simulink model "Quadroto_Outer_Loop"  (Simulink 7.6)
settings: Solver=FixedStepDiscrete  StartTime=0.0  StopTime=10.0  FixedStep=0.01  RelTol=1e-3
libraries: passive_control x1
settings Model: Creator=jporter  LastModifiedBy=Administrator
settings DataIOCC: LimitDataPoints=off  SaveOutput=off  SignalLogging=off  DSMLogging=off  SaveTime=off
settings OptimizationCC: InlineParams=on  EnhancedBackFolding=on  PassReuseOutputArgsAs=Individual arguments  OptimizeModelRefInitCode=on
settings HardwareCC: ProdLargestAtomicInteger=Long  ProdLargestAtomicFloat=Float  ProdIntDivRoundTo=Floor  ProdEndianess=LittleEndian  ProdHWDeviceType=ARM Compatible->ARM 7  TargetLargestAtomicInteger=Long  TargetLargestAtomicFloat=Float  TargetIntDivRoundTo=Floor  TargetEndianess=LittleEndian  TargetHWDeviceType=ARM Compatible->ARM 7
settings RTWCC: SystemTargetFile=ert.tlc  GenCodeOnly=on  TemplateMakefile=ert_default_tmf  Description=Real-Time Workshop Embedded Coder  GenerateReport=on  ProcessScript=ert_make_rtw_hook  IncludeHyperlinkInReport=on  LaunchReport=on  GenerateTraceReportSl=on  GenerateTraceReportEml=on  RTWCompilerOptimization=On  CheckMdlBeforeBuild=Warning
settings CodeAppCC: IgnoreCustomStorageClasses=off
settings ERTTargetCC: MultiwordLength=2048  GenerateSampleERTMain=on  CombineSignalStateStructs=on  MultiInstanceERTCode=on  SupportComplex=off  MultiInstanceErrorCode=Warning  ERTCustomFileTemplate=example_file_process.tlc

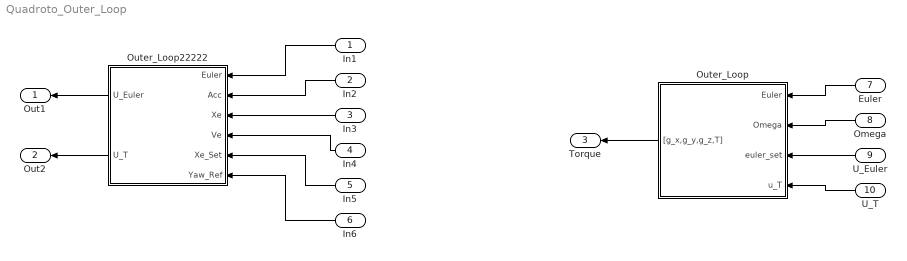
== system Quadroto_Outer_Loop ==
  In1 : Inport  OutDataTypeStr=single  PortDimensions=[3]
  In2 : Inport  Port=2  OutDataTypeStr=single  PortDimensions=[3]
  In3 : Inport  Port=3  OutDataTypeStr=single  PortDimensions=[3]
  In4 : Inport  Port=4  OutDataTypeStr=single  PortDimensions=[3]
  In5 : Inport  Port=5  OutDataTypeStr=single  PortDimensions=[3]
  In6 : Inport  Port=6  OutDataTypeStr=single  PortDimensions=[1]
  Euler : Inport  Port=7  OutDataTypeStr=single  PortDimensions=[3]
  Omega : Inport  Port=8  OutDataTypeStr=single  PortDimensions=[3]
  U_Euler : Inport  Port=9  OutDataTypeStr=single  PortDimensions=[3]
  U_T : Inport  Port=10  OutDataTypeStr=single  PortDimensions=[1]
  Outer_Loop : Subsystem
  Outer_Loop22222 : Subsystem
  Out1 : Outport
  Out2 : Outport  Port=2
  Torque : Outport  Port=3
  wires:
  In1/1 -> Outer_Loop22222/1(Euler)
  In2/1 -> Outer_Loop22222/2(Acc)
  In3/1 -> Outer_Loop22222/3(Xe)
  In4/1 -> Outer_Loop22222/4(Ve)
  In5/1 -> Outer_Loop22222/5(Xe_Set)
  In6/1 -> Outer_Loop22222/6(Yaw_Ref)
  Outer_Loop22222/1(U_Euler) -> Out1/1
  Outer_Loop22222/2(U_T) -> Out2/1
  Euler/1 -> Outer_Loop/1(Euler)
  Omega/1 -> Outer_Loop/2(Omega)
  U_Euler/1 -> Outer_Loop/3(euler_set)
  U_T/1 -> Outer_Loop/4(u_T)
  Outer_Loop/1("[g_x,g_y,g_z,T]") -> Torque/1

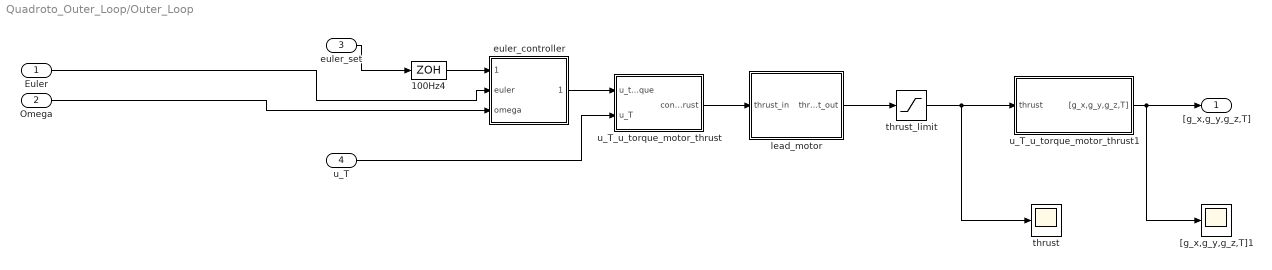
== system Quadroto_Outer_Loop/Outer_Loop ==
  Euler : Inport  OutDataTypeStr=single
  Omega : Inport  Port=2  OutDataTypeStr=single
  euler_set : Inport  Port=3  OutDataTypeStr=single
  u_T : Inport  Port=4  OutDataTypeStr=single
  100Hz4 : ZeroOrderHold  SampleTime=.01
  "[g_x,g_y,g_z,T]1" : Scope
      settings: TimeRange=100  YMin=3  YMax=10  SaveName=thrust_data10  MaxDataPoints=50000
  euler_controller : Subsystem  mask{K=1, K_e=2*7.5/.65, K_o=.5*.25, I=diag([2.32,2.32,4.41]*1e-3), T_max=3.7*1, delta=.343/2, K_t=1.5e-9/6.11e-8}
      mask prompts: K "Loop Gain [K]:"; K_e "Euler Gain [K_e]:"; K_o "Omega Gain [K_o]:"; I "Inertia Matrix [I]:"; T_max "Max Rotor Thrust [T_max] (N):"; delta "Distance from CG to rotor [delta] (m):"; K_t "z-torque gain [K_t]:"
      mask init:
      | I=[I(1,1),I(2,2),I(3,3)];
      | I_norm=I*(1/min(I))
  lead_motor : Subsystem  mask{tau_motor=1/20, Ts=1/100, m=.489}
      mask prompts: m "mass of quadrotor (kg) [m]"
      mask init:
      | Hs=tf([tau_motor, 1],[Ts/pi, 1]);
      | Hz=ipesh_transform(Hs,Ts)
      | Hz.num{1}
      | Hz.den{1}
      | %a=1/tau_motor;
      | %b=pi/t_s;
      | %T=t_s;
      | %num1=b*(1-exp(-b*T))+a*(b*T-1+exp(-b*T));
      | %num2=-b*(1-exp(-b*T))+a*(1-exp(-b*T)-b*T*exp(-b*T));
      | %den1=a*b;
      | %den2=-a*b*exp(-b*T);
      | %num=[num1 num2];
      | %den=[den1 den2];
      | %Hz=tf(num,den,T);
      | %[y,t]=step(Hz);
      | %k_ss=(1/y(length(y)));
      | %num=k_ss*num;
      | %lead_a_1=single(-den(2)/den(1))
      | %lead_b_1=single(num(2)/den(1))
      | %lead_b_2=single(num(1)/den(1))
      | %Hz=k_ss*Hz
      | %bode(Hz);
  thrust : Scope
      settings: TimeRange=100  YMin=3  YMax=10  SaveName=thrust_data  MaxDataPoints=50000
  thrust_limit : Saturate  UpperLimit=3.7*ones(4,1)  LowerLimit=0*ones(4,1)  OutDataTypeStr=single
  u_T_u_torque_motor_thrust : Subsystem  mask{dx=1*.343/2, K_torque=1.5e-9/6.11e-8}
      mask prompts: dx "X distance of motor from CG [dx](meters):"; K_torque "Ktorque [K_torque]:"
      mask init:
      | M=[0 -dx 0 dx;
      |    dx 0 -dx 0;
      |    -K_torque K_torque -K_torque K_torque;
      |    1 1 1 1];
      | Mi=single(inv(M))
  u_T_u_torque_motor_thrust1 : Subsystem  mask{delta=.343/2, K_t=1.5e-9/6.11e-8, T_max=3.7, Ts=.01}
      mask prompts: delta "X distance of motor from CG [delta](meters):"; K_t "Ktorque [K_torque]:"; T_max "Max Rotor Thrust [T_max]:"; Ts "Sample Time [Ts]:"
      mask init:
      | M=single([0 -delta 0 delta;
      |    delta 0 -delta 0;
      |    -K_t K_t -K_t K_t;
      |    1 1 1 1]);
  "[g_x,g_y,g_z,T]" : Outport
  wires:
  euler_set/1 -> 100Hz4/1
  u_T/1 -> u_T_u_torque_motor_thrust/2(u_T)
  euler_controller/1(u_torque) -> u_T_u_torque_motor_thrust/1(u_torque)
  thrust_limit/1 -> thrust/1, u_T_u_torque_motor_thrust1/1(thrust)
  u_T_u_torque_motor_thrust/1(cont_motor_thrust) -> lead_motor/1(thrust_in)
  lead_motor/1(thrust_out) -> thrust_limit/1
  u_T_u_torque_motor_thrust1/1("[g_x,g_y,g_z,T]") -> "[g_x,g_y,g_z,T]"/1, "[g_x,g_y,g_z,T]1"/1
  100Hz4/1 -> euler_controller/1(euler_set)
  Euler/1 -> euler_controller/2(euler)
  Omega/1 -> euler_controller/3(omega)

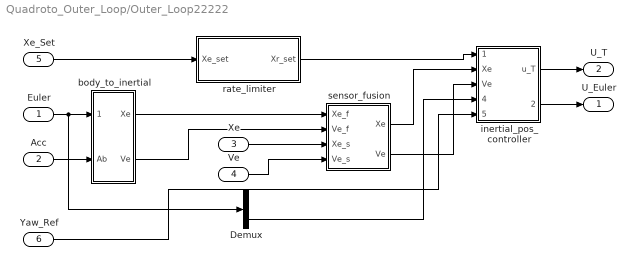
== system Quadroto_Outer_Loop/Outer_Loop22222 ==
  Euler : Inport  OutDataTypeStr=single  PortDimensions=[3]
  Acc : Inport  Port=2  OutDataTypeStr=single  PortDimensions=[3]
  Xe : Inport  Port=3  OutDataTypeStr=single  PortDimensions=[3]
  Ve : Inport  Port=4  OutDataTypeStr=single  PortDimensions=[3]
  Xe_Set : Inport  Port=5  OutDataTypeStr=single  PortDimensions=[3]
  Yaw_Ref : Inport  Port=6  OutDataTypeStr=single  PortDimensions=[1]
  Demux : Demux  Outputs=3
  body_to_inertial : Subsystem
  inertial_pos_controller : Subsystem
  rate_limiter : Subsystem  mask{wn=2*pi, zeta=0.9, Vmax=2, T=0.01}
      mask prompts: wn "omega_n"; Vmax "Max velocity"; T "Sample time"
      mask init:
      | Hs=tf([wn^2],[1,2*zeta*wn,wn^2]);
      | Hz=ipesh_transform(Hs,T);
  sensor_fusion : Subsystem  mask{tau=.1, Ts=.01, Ts_gps=.1}
      mask prompts: tau "low-pass time constant (sec) [tau]"; Ts "Sample time [Ts]"; Ts_gps "GPS Sample Time [Ts_gps]"
  U_Euler : Outport  OutDataTypeStr=single  PortDimensions=[3]
  U_T : Outport  Port=2  OutDataTypeStr=single  PortDimensions=[1]
  wires:
  Xe_Set/1 -> rate_limiter/1(Xe_set)
  inertial_pos_controller/1(u_T) -> U_T/1
  inertial_pos_controller/2(u_euler) -> U_Euler/1
  Euler/1 -> body_to_inertial/1(euler), Demux/1
  Acc/1 -> body_to_inertial/2(Ab)
  sensor_fusion/1(Xe) -> inertial_pos_controller/2(Xe)
  sensor_fusion/2(Ve) -> inertial_pos_controller/3(Ve)
  body_to_inertial/1(Xe) -> sensor_fusion/1(Xe_f)
  body_to_inertial/2(Ve) -> sensor_fusion/2(Ve_f)
  Xe/1 -> sensor_fusion/3(Xe_s)
  Ve/1 -> sensor_fusion/4(Ve_s)
  rate_limiter/1(Xr_set) -> inertial_pos_controller/1(Xe_set)
  Demux/3 -> inertial_pos_controller/4(Yaw_actual)
  Yaw_Ref/1 -> inertial_pos_controller/5(Yaw_set)

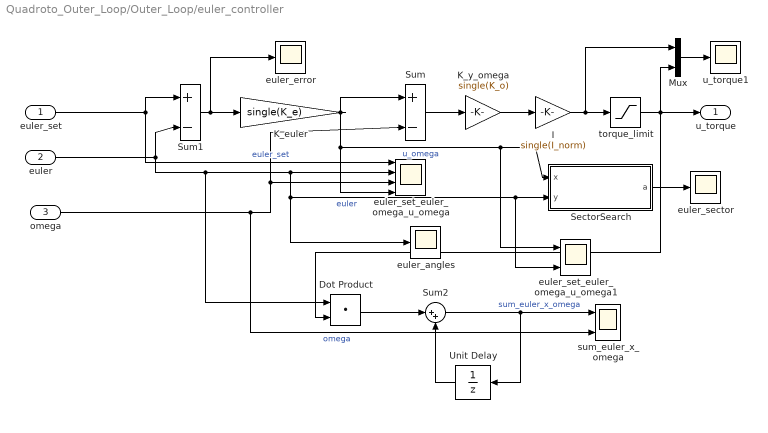
== system Quadroto_Outer_Loop/Outer_Loop/euler_controller ==
  euler_set : Inport
  euler : Inport  Port=2
  omega : Inport  Port=3
  Dot Product : DotProduct  InputSameDT=on  OutDataTypeStr=Inherit: Inherit via internal rule
  I : Gain  Gain=single(I_norm)  OutDataTypeStr=single
  K_euler : Gain  Gain=single(K_e)
  K_y_omega : Gain  Gain=single(K_o)  OutDataTypeStr=single
  Mux : Mux  Inputs=2
  SectorSearch : Subsystem  AncestorBlock=passive_control/SectorSearch
  Sum : Sum  Inputs=|+-  AccumDataTypeStr=single
  Sum1 : Sum  Inputs=|+-  AccumDataTypeStr=single
  Sum2 : Sum  Inputs=|++
  Unit Delay : UnitDelay  SampleTime=-1
  euler_angles : Scope
      settings: TimeRange=80  YMin=-1.1  YMax=1.1  SaveName=euler_data  MaxDataPoints=50000
  euler_error : Scope
      settings: TimeRange=80  YMin=-0.011  YMax=0.011  SaveName=euler_data1  MaxDataPoints=50000
  euler_sector : Scope
      settings: TimeRange=80  YMin=-1  YMax=1  SaveName=euler_sector_data  MaxDataPoints=50000
  euler_set_euler_omega_u_omega : Scope  NumInputPorts=4
      settings: YMin=-7~-7~-0.3~-0.3  YMax=1~1~0.3~0.3  SaveName=ScopeData8
  euler_set_euler_omega_u_omega1 : Scope  NumInputPorts=2
      settings: YMin=-7~-7  YMax=1~1  SaveName=ScopeData5  Decimation=10
  sum_euler_x_omega : Scope  NumInputPorts=2
      settings: YMin=-0.5~-5  YMax=2~5  SaveName=ScopeData6  Decimation=20
  torque_limit : Saturate  UpperLimit=[delta,delta,2*K_t]*T_max  LowerLimit=-[delta,delta,2*K_t]*T_max  OutDataTypeStr=single
  u_torque1 : Scope
      settings: TimeRange=80  YMin=-1  YMax=1  SaveName=euler_sector_data1  MaxDataPoints=50000
  u_torque : Outport
  wires:
  Sum/1 -> K_y_omega/1
  euler_set/1 -> Sum1/1, euler_set_euler_omega_u_omega/1  "euler_set"
  Sum1/1 -> K_euler/1, euler_error/1
  euler/1 -> Sum1/2, euler_set_euler_omega_u_omega/2, SectorSearch/2(y), euler_set_euler_omega_u_omega1/2, euler_angles/1, Dot Product/1  "euler"
  K_euler/1 -> euler_set_euler_omega_u_omega/4, SectorSearch/1(x), euler_set_euler_omega_u_omega1/1, Sum/1  "u_omega"
  torque_limit/1 -> u_torque/1, Dot Product/2, Mux/2
  K_y_omega/1 -> I/1
  omega/1 -> Sum/2, euler_set_euler_omega_u_omega/3, sum_euler_x_omega/2  "omega"
  SectorSearch/1(a) -> euler_sector/1
  Sum2/1 -> sum_euler_x_omega/1, Unit Delay/1  "sum_euler_x_omega"
  Unit Delay/1 -> Sum2/2
  Dot Product/1 -> Sum2/1
  I/1 -> torque_limit/1, Mux/1
  Mux/1 -> u_torque1/1

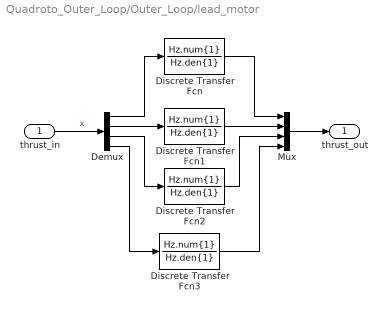
== system Quadroto_Outer_Loop/Outer_Loop/lead_motor ==
  thrust_in : Inport  OutDataTypeStr=single
  Demux : Demux
  Discrete Transfer Fcn{,1..3} (4 alike) : DiscreteTransferFcn  Numerator=Hz.num{1}  Denominator=Hz.den{1}  InitialStates=9.81*m/4  SampleTime=-1
  Mux : Mux
  thrust_out : Outport  OutDataTypeStr=single
  wires:
  thrust_in/1 -> Demux/1  "x"
  Demux/1 -> Discrete Transfer Fcn/1
  Demux/2 -> Discrete Transfer Fcn1/1
  Demux/3 -> Discrete Transfer Fcn2/1
  Mux/1 -> thrust_out/1
  Discrete Transfer Fcn/1 -> Mux/1
  Discrete Transfer Fcn1/1 -> Mux/2
  Discrete Transfer Fcn2/1 -> Mux/3
  Demux/4 -> Discrete Transfer Fcn3/1
  Discrete Transfer Fcn3/1 -> Mux/4

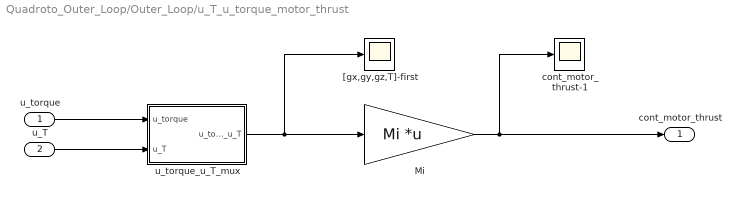
== system Quadroto_Outer_Loop/Outer_Loop/u_T_u_torque_motor_thrust ==
  u_torque : Inport
  u_T : Inport  Port=2
  Mi : Gain  Gain=Mi  Multiplication=Matrix(K*u)  ParamDataTypeStr=single  OutDataTypeStr=single
  "[gx,gy,gz,T]-first" : Scope
      settings: TimeRange=100  YMin=3  YMax=10  SaveName=thrust_data6  MaxDataPoints=50000
  cont_motor_thrust-1 : Scope
      settings: TimeRange=100  YMin=3  YMax=10  SaveName=thrust_data7  MaxDataPoints=50000
  u_torque_u_T_mux : Stateflow chart  TreatAsAtomicUnit=on
  cont_motor_thrust : Outport
  wires:
  u_torque/1 -> u_torque_u_T_mux/1(u_torque)
  u_T/1 -> u_torque_u_T_mux/2(u_T)
  Mi/1 -> cont_motor_thrust/1, cont_motor_thrust-1/1
  u_torque_u_T_mux/1(u_torque_u_T) -> Mi/1, "[gx,gy,gz,T]-first"/1

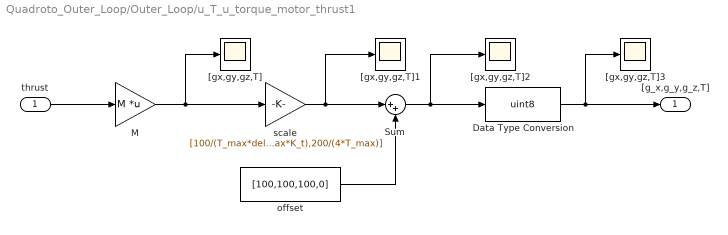
== system Quadroto_Outer_Loop/Outer_Loop/u_T_u_torque_motor_thrust1 ==
  thrust : Inport
  Data Type Conversion : DataTypeConversion  OutMin=[0]  OutMax=[200]  OutDataTypeStr=uint8  SaturateOnIntegerOverflow=on
  M : Gain  Gain=M  Multiplication=Matrix(K*u)  ParamDataTypeStr=single  OutDataTypeStr=single
  Sum : Sum  Inputs=|++
  [gx,gy,gz,T]{,1..3} (4 alike) : Scope
      "[gx,gy,gz,T]" settings: TimeRange=100  YMin=3  YMax=10  SaveName=thrust_data4  MaxDataPoints=50000
      "[gx,gy,gz,T]1" settings: TimeRange=100  YMin=3  YMax=10  SaveName=thrust_data5  MaxDataPoints=50000
      "[gx,gy,gz,T]2" settings: TimeRange=100  YMin=3  YMax=10  SaveName=thrust_data8  MaxDataPoints=50000
      "[gx,gy,gz,T]3" settings: TimeRange=100  YMin=3  YMax=10  SaveName=thrust_data9  MaxDataPoints=50000
  offset : Constant  Value=[100,100,100,0]  SampleTime=Ts
  scale : Gain  Gain=[100/(T_max*delta),-100/(T_max*delta),-100/(2*T_max*K_t),200/(4*T_max)]  ParamDataTypeStr=single  OutDataTypeStr=single
  "[g_x,g_y,g_z,T]" : Outport
  wires:
  M/1 -> scale/1, "[gx,gy,gz,T]"/1
  thrust/1 -> M/1
  scale/1 -> Sum/1, "[gx,gy,gz,T]1"/1
  Sum/1 -> Data Type Conversion/1, "[gx,gy,gz,T]2"/1
  offset/1 -> Sum/2
  Data Type Conversion/1 -> "[g_x,g_y,g_z,T]"/1, "[gx,gy,gz,T]3"/1

== system Quadroto_Outer_Loop/Outer_Loop22222/body_to_inertial ==
  euler : Inport
  Ab : Inport  Port=2
  Ab_to_Ae : Stateflow chart  TreatAsAtomicUnit=on
  inertial_vel_and pos_est : Subsystem  mask{Ts=.01}
      mask prompts: Ts "Sample Time [Ts] (seconds):"
  Xe : Outport
  Ve : Outport  Port=2
  wires:
  euler/1 -> Ab_to_Ae/1(euler)
  Ab/1 -> Ab_to_Ae/2(Ab)
  Ab_to_Ae/1(Ae) -> inertial_vel_and pos_est/1(Ab)
  inertial_vel_and pos_est/1(Vb) -> Ve/1
  inertial_vel_and pos_est/2(Xb) -> Xe/1

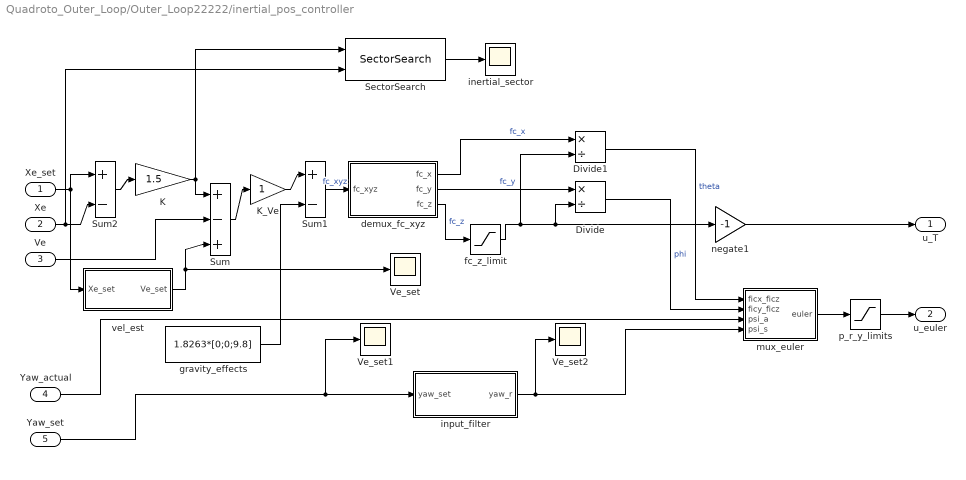
== system Quadroto_Outer_Loop/Outer_Loop22222/inertial_pos_controller ==
  Xe_set : Inport
  Xe : Inport  Port=2
  Ve : Inport  Port=3
  Yaw_actual : Inport  Port=4
  Yaw_set : Inport  Port=5
  Divide : Product  Inputs=*/  OutDataTypeStr=single
  Divide1 : Product  Inputs=*/  OutDataTypeStr=single
  K : Gain  Gain=1.5  OutDataTypeStr=single
  K_Ve : Gain  ParamDataTypeStr=single  OutDataTypeStr=single
  SectorSearch : passive_control/SectorSearch  SystemSampleTime=-1
  Sum : Sum  Inputs=|+-+  AccumDataTypeStr=single  OutDataTypeStr=single
  Sum1 : Sum  Inputs=|+-  AccumDataTypeStr=single  OutDataTypeStr=single
  Sum2 : Sum  Inputs=|+-  AccumDataTypeStr=single  OutDataTypeStr=single
  Ve_set : Scope
      settings: TimeRange=60  YMin=-1.75  YMax=2.25  SaveName=ScopeData2  Decimation=10
  Ve_set1 : Scope
      settings: TimeRange=60  SaveName=ScopeData10  Decimation=10
  Ve_set2 : Scope
      settings: TimeRange=60  SaveName=ScopeData11  Decimation=10
  demux_fc_xyz : Stateflow chart  TreatAsAtomicUnit=on
  fc_z_limit : Saturate  UpperLimit=-(1/8)*9.81  LowerLimit=-4*9.81  OutDataTypeStr=single
  gravity_effects : Constant  Value=1.8263*[0;0;9.8]  OutDataTypeStr=single
  inertial_sector : Scope
      settings: TimeRange=80  YMin=-1  YMax=1  SaveName=inertial_sector_data  MaxDataPoints=50000
  input_filter : Subsystem  mask{wn=1, zeta=0.9, T=0.01}
      mask prompts: wn "omega_n"; T "Sample time"
      mask init:
      | Hs=tf([wn^2],[1,2*zeta*wn,wn^2]);
      | Hz=ipesh_transform(Hs,T);
  mux_euler : Stateflow chart  TreatAsAtomicUnit=on
  negate1 : Gain  Gain=-1  OutDataTypeStr=single
  p_r_y_limits : Saturate  UpperLimit=[pi/4,pi/4,inf]  LowerLimit=-[pi/4,pi/4,inf]  OutDataTypeStr=single
  vel_est : Subsystem  mask{tau_f=.01/pi, T=.01}
      mask prompts: T "sample rate"
      mask init:
      | %b=1/tau_f;
      | %num1=(1-exp(-b*T));
      | %num2=-num1;
      | %den1=1;
      | %den2=-exp(-b*T);
      | %num=(1/T)*[num1 num2];
      | %den=[den1 den2];
      | %vel_est_a_1=single(-den(2)/den(1))
      | %vel_est_b_1=single(num(2)/den(1))
      | %vel_est_b_2=single(num(1)/den(1))
      | Hs=tf([1 0],[T/pi 1]);
      | Hz=ipesh_transform(Hs,T);
      | %Hz=tf(num,den,T);
      | %bode(Hz);
      | %hold on;
      | %bode(tf([1 0],[tau_f 1]));
  u_T : Outport
  u_euler : Outport  Port=2
  wires:
  fc_z_limit/1 -> Divide1/2, Divide/2, negate1/1
  Xe_set/1 -> Sum2/1, vel_est/1(Xe_set)
  negate1/1 -> u_T/1
  p_r_y_limits/1 -> u_euler/1
  demux_fc_xyz/1(fc_x) -> Divide1/1  "fc_x"
  demux_fc_xyz/3(fc_z) -> fc_z_limit/1  "fc_z"
  mux_euler/1(euler) -> p_r_y_limits/1
  Sum1/1 -> demux_fc_xyz/1(fc_xyz)  "fc_xyz"
  gravity_effects/1 -> Sum1/2
  Sum/1 -> K_Ve/1
  Xe/1 -> Sum2/2, SectorSearch/2
  Sum2/1 -> K/1
  K/1 -> Sum/1, SectorSearch/1
  demux_fc_xyz/2(fc_y) -> Divide/1  "fc_y"
  K_Ve/1 -> Sum1/1
  Ve/1 -> Sum/2
  vel_est/1(Ve_set) -> Sum/3, Ve_set/1
  Divide1/1 -> mux_euler/1(ficx_ficz)  "theta"
  Divide/1 -> mux_euler/2(ficy_ficz)  "phi"
  input_filter/1(yaw_r) -> Ve_set2/1, mux_euler/4(psi_s)
  Yaw_set/1 -> input_filter/1(yaw_set), Ve_set1/1
  Yaw_actual/1 -> mux_euler/3(psi_a)
  SectorSearch/1 -> inertial_sector/1

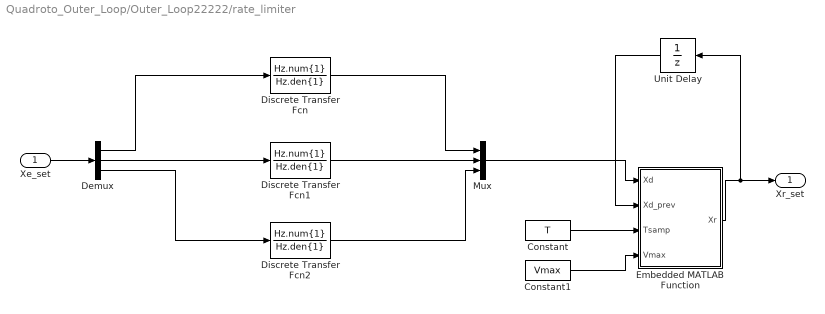
== system Quadroto_Outer_Loop/Outer_Loop22222/rate_limiter ==
  Xe_set : Inport
  Constant : Constant  Value=T  OutDataTypeStr=single
  Constant1 : Constant  Value=Vmax  OutDataTypeStr=single
  Demux : Demux  Outputs=3
  Discrete Transfer Fcn : DiscreteTransferFcn  Numerator=Hz.num{1}  Denominator=Hz.den{1}  SampleTime=-1
  Discrete Transfer Fcn1 : DiscreteTransferFcn  Numerator=Hz.num{1}  Denominator=Hz.den{1}  SampleTime=-1
  Discrete Transfer Fcn2 : DiscreteTransferFcn  Numerator=Hz.num{1}  Denominator=Hz.den{1}  SampleTime=-1
  Embedded MATLAB Function : Stateflow chart  TreatAsAtomicUnit=on
  Mux : Mux  Inputs=3
  Unit Delay : UnitDelay  SampleTime=-1
  Xr_set : Outport
  wires:
  Xe_set/1 -> Demux/1
  Mux/1 -> Embedded MATLAB Function/1(Xd)
  Embedded MATLAB Function/1(Xr) -> Xr_set/1, Unit Delay/1
  Unit Delay/1 -> Embedded MATLAB Function/2(Xd_prev)
  Constant/1 -> Embedded MATLAB Function/3(Tsamp)
  Constant1/1 -> Embedded MATLAB Function/4(Vmax)
  Demux/1 -> Discrete Transfer Fcn/1
  Discrete Transfer Fcn/1 -> Mux/1
  Demux/2 -> Discrete Transfer Fcn1/1
  Discrete Transfer Fcn1/1 -> Mux/2
  Demux/3 -> Discrete Transfer Fcn2/1
  Discrete Transfer Fcn2/1 -> Mux/3

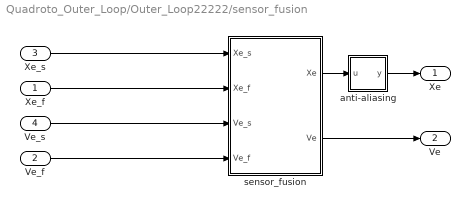
== system Quadroto_Outer_Loop/Outer_Loop22222/sensor_fusion ==
  Xe_f : Inport
  Ve_f : Inport  Port=2
  Xe_s : Inport  Port=3
  Ve_s : Inport  Port=4
  anti-aliasing : Subsystem  mask{tau=tau, Ts=Ts}
      mask prompts: tau "tau (sec)"; Ts "Ts (sec)"
      mask init:
      | Hs = tf(1,[tau,1]);
      | Hz = ipesh_transform(Hs,Ts);
  sensor_fusion : Stateflow chart  TreatAsAtomicUnit=on
  Xe : Outport
  Ve : Outport  Port=2
  wires:
  Xe_f/1 -> sensor_fusion/2(Xe_f)
  Ve_f/1 -> sensor_fusion/4(Ve_f)
  sensor_fusion/1(Xe) -> anti-aliasing/1(u)
  anti-aliasing/1(y) -> Xe/1
  Xe_s/1 -> sensor_fusion/1(Xe_s)
  sensor_fusion/2(Ve) -> Ve/1
  Ve_s/1 -> sensor_fusion/3(Ve_s)

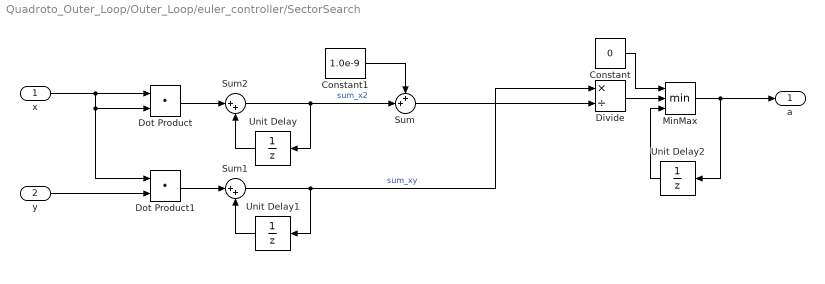
== system Quadroto_Outer_Loop/Outer_Loop/euler_controller/SectorSearch ==
  x : Inport
  y : Inport  Port=2
  Constant : Constant  Value=0
  Constant1 : Constant  Value=1.0e-9
  Divide : Product  Inputs=*/
  Dot Product : DotProduct  InputSameDT=on  OutDataTypeStr=Inherit: Inherit via internal rule
  Dot Product1 : DotProduct  InputSameDT=on  OutDataTypeStr=Inherit: Inherit via internal rule
  MinMax : MinMax  Inputs=3
  Sum : Sum  Inputs=++|
  Sum1 : Sum  Inputs=|++
  Sum2 : Sum  Inputs=|++
  Unit Delay : UnitDelay  SampleTime=-1
  Unit Delay1 : UnitDelay  SampleTime=-1
  Unit Delay2 : UnitDelay  SampleTime=-1
  a : Outport
  wires:
  Constant1/1 -> Sum/1
  Sum/1 -> Divide/2
  Unit Delay2/1 -> MinMax/3
  Divide/1 -> MinMax/2
  Constant/1 -> MinMax/1
  MinMax/1 -> a/1, Unit Delay2/1
  y/1 -> Dot Product1/2
  x/1 -> Dot Product1/1, Dot Product/2, Dot Product/1
  Dot Product1/1 -> Sum1/1
  Unit Delay1/1 -> Sum1/2
  Sum1/1 -> Divide/1, Unit Delay1/1  "sum_xy"
  Dot Product/1 -> Sum2/1
  Unit Delay/1 -> Sum2/2
  Sum2/1 -> Sum/2, Unit Delay/1  "sum_x2"

== system Quadroto_Outer_Loop/Outer_Loop22222/body_to_inertial/inertial_vel_and pos_est ==
  Ab : Inport
  DT_integrator : Subsystem
  DT_integrator1 : Subsystem
  Vb : Outport
  Xb : Outport  Port=2
  wires:
  DT_integrator1/1(Xb) -> Xb/1
  Ab/1 -> DT_integrator/1(Ab)
  DT_integrator/1(Vb) -> Vb/1, DT_integrator1/1(Vb)

== system Quadroto_Outer_Loop/Outer_Loop22222/inertial_pos_controller/input_filter ==
  yaw_set : Inport
  Discrete Transfer Fcn : DiscreteTransferFcn  Numerator=Hz.num{1}  Denominator=Hz.den{1}  SampleTime=-1
  yaw_r : Outport
  wires:
  yaw_set/1 -> Discrete Transfer Fcn/1
  Discrete Transfer Fcn/1 -> yaw_r/1

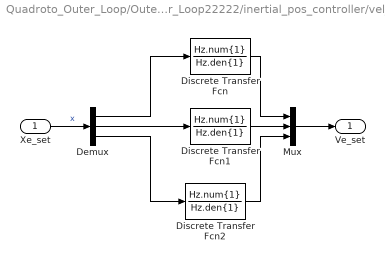
== system Quadroto_Outer_Loop/Outer_Loop22222/inertial_pos_controller/vel_est ==
  Xe_set : Inport
  Demux : Demux  Outputs=3
  Discrete Transfer Fcn : DiscreteTransferFcn  Numerator=Hz.num{1}  Denominator=Hz.den{1}  SampleTime=-1
  Discrete Transfer Fcn1 : DiscreteTransferFcn  Numerator=Hz.num{1}  Denominator=Hz.den{1}  SampleTime=-1
  Discrete Transfer Fcn2 : DiscreteTransferFcn  Numerator=Hz.num{1}  Denominator=Hz.den{1}  SampleTime=-1
  Mux : Mux  Inputs=3
  Ve_set : Outport
  wires:
  Xe_set/1 -> Demux/1  "x"
  Demux/1 -> Discrete Transfer Fcn/1
  Demux/2 -> Discrete Transfer Fcn1/1
  Demux/3 -> Discrete Transfer Fcn2/1
  Mux/1 -> Ve_set/1
  Discrete Transfer Fcn/1 -> Mux/1
  Discrete Transfer Fcn1/1 -> Mux/2
  Discrete Transfer Fcn2/1 -> Mux/3

== system Quadroto_Outer_Loop/Outer_Loop22222/sensor_fusion/anti-aliasing ==
  u : Inport
  Demux : Demux  Outputs=3
  Mux : Mux  Inputs=3
  smoothing-filter : DiscreteTransferFcn  Numerator=Hz.num{1}  Denominator=Hz.den{1}  SampleTime=-1
  smoothing-filter1 : DiscreteTransferFcn  Numerator=Hz.num{1}  Denominator=Hz.den{1}  SampleTime=-1
  y : Outport
  wires:
  Demux/3 -> Mux/3
  Demux/2 -> smoothing-filter1/1
  smoothing-filter1/1 -> Mux/2
  smoothing-filter/1 -> Mux/1
  Demux/1 -> smoothing-filter/1
  Mux/1 -> y/1
  u/1 -> Demux/1

== system Quadroto_Outer_Loop/Outer_Loop22222/body_to_inertial/inertial_vel_and pos_est/DT_integrator ==
  Ab : Inport
  Sum : Sum  Inputs=++|  OutDataTypeStr=single
  Sum1 : Sum  Inputs=|++  AccumDataTypeStr=single
  negate : Gain  Gain=.5*Ts  OutDataTypeStr=single
  u_delay : UnitDelay  SampleTime=-1
  u_delay1 : UnitDelay  SampleTime=-1
  Vb : Outport
  wires:
  Ab/1 -> u_delay/1, Sum/2
  u_delay/1 -> Sum/1
  Sum/1 -> negate/1
  negate/1 -> Sum1/1
  Sum1/1 -> u_delay1/1, Vb/1
  u_delay1/1 -> Sum1/2

== system Quadroto_Outer_Loop/Outer_Loop22222/body_to_inertial/inertial_vel_and pos_est/DT_integrator1 ==
  Vb : Inport
  Sum : Sum  Inputs=++|  OutDataTypeStr=single
  Sum1 : Sum  Inputs=|++  OutDataTypeStr=single
  negate : Gain  Gain=.5*Ts  OutDataTypeStr=single
  u_delay : UnitDelay  SampleTime=-1
  u_delay1 : UnitDelay  SampleTime=-1
  Xb : Outport  OutDataTypeStr=single  PortDimensions=[3]
  wires:
  u_delay1/1 -> Sum1/2
  Sum1/1 -> Xb/1, u_delay1/1
  negate/1 -> Sum1/1
  Sum/1 -> negate/1
  u_delay/1 -> Sum/1
  Vb/1 -> Sum/2, u_delay/1

== matlab function Outer_Loop22222/body_to_inertial/Ab_to_Ae ==
  data: euler input single size=[3]; Ae output single size=[3]; Ab input single size=[3]
function Ae = fcn(euler, Ab)
% This block supports the Embedded MATLAB subset.
% See the help menu for details. 
phi=euler(1);
theta=euler(2);
psi=euler(3);
c_phi=cos(phi);
c_theta=cos(theta);
c_psi=cos(psi);
s_phi=sin(phi);
s_theta=sin(theta);
s_psi=sin(psi);
R=single([c_theta*c_psi, c_theta*s_psi, -s_theta;
   s_phi*s_theta*c_psi-c_phi*s_psi, s_phi*s_theta*s_psi+c_phi*c_psi, c_theta*s_phi;
   c_phi*s_theta*c_psi+s_phi*s_psi, c_phi*s_theta*s_psi-s_phi*c_psi, c_theta*c_phi]);
%R=single(zeros(3,3));
%R(1,1)=c_theta*c_psi;
%R(1,2)=c_theta*s_psi;
%R(1,3)=-s_theta;
%R(2,1)=s_phi*s_theta*c_psi - c_phi*s_psi;
%R(2,2)=s_phi*s_theta*s_psi + c_phi*c_psi;
%R(2,3)=c_theta*s_phi;
%R(3,1)=c_phi*s_theta*c_psi + s_phi*s_psi;
%R(3,2)=c_phi*s_theta*s_psi - s_phi*c_psi;
%R(3,3)=c_theta*c_phi;
Ae= transpose(R) * Ab;
%Ae= single(Aed);

== matlab function Outer_Loop/u_T_u_torque_motor_thrust/u_torque_u_T_mux ==
  data: u_torque input single size=[3]; u_torque_u_T output single size=[4]; u_T input single size=[1]
function u_torque_u_T = fcn(u_torque, u_T)
% This block supports the Embedded MATLAB subset.
% See the help menu for details. 
u_torque_u_T = [u_torque; u_T];

== matlab function Outer_Loop22222/inertial_pos_controller/demux_fc_xyz ==
  data: fc_xyz input single size=[3]; fc_x output single size=[1]; fc_y output single size=[1]; fc_z output single size=[1]
function [fc_x,fc_y, fc_z] = fcn(fc_xyz)
% This block supports the Embedded MATLAB subset.
% See the help menu for details. 
fc_x=fc_xyz(1);
fc_y=fc_xyz(2);
fc_z=fc_xyz(3);

== matlab function Outer_Loop22222/inertial_pos_controller/mux_euler ==
  data: ficx_ficz input single size=[1]; euler output single size=[3]; ficy_ficz input single size=[1]; psi_a input single size=[1]; psi_s input single
function euler = fcn(ficx_ficz, ficy_ficz, psi_a, psi_s)
% This block supports the Embedded MATLAB subset.
% See the help menu for details. 

A = [sin(psi_a) -cos(psi_a); cos(psi_a) sin(psi_a)];
% Get [phi, theta] 
euler_angs = (A * [ficx_ficz; ficy_ficz])';

euler=[euler_angs(1);euler_angs(2);psi_s];

== matlab function Outer_Loop22222/rate_limiter/Embedded MATLAB Function ==
  data: Xd input single; Xr output single; Xd_prev input single; Tsamp input single; Vmax input single
function Xr = limit_rate(Xd, Xd_prev, Tsamp, Vmax)
% This block supports the Embedded MATLAB subset.
% See the help menu for details. 

delta = Xd - Xd_prev;
delta = sign(delta) .* min( abs(delta), (ones(size(delta)) * Tsamp * Vmax) );

Xr = Xd_prev + delta;

== matlab function Outer_Loop22222/sensor_fusion/sensor_fusion ==
  data: Xe_s input double; Xe output double; Xe_f input double; Ve_s input double; Ve_f input double; Ve output double; Ts_gps parameter double; Ts parameter double
function [Xe,Ve] = fcn(Xe_s, Xe_f, Ve_s, Ve_f, Ts_gps, Ts)
%Fuse the gps measurements Xe_s and Ve_s with the
%faster inertial sensor measurements Xe_f, Ve_f
%N.B. the height is updated by a fast pressure sensor so we always
%pass through the z-component of Xe_s and Ve_s
persistent count;
persistent dXe_s_last;
persistent dVe_s_last;
persistent dXe_s_last_2;
if isempty(count)
    count = floor(Ts_gps/Ts);
    dXe_s_last = Xe_s-Xe_f;
    dXe_s_last_2 = dXe_s_last;
    dVe_s_last = Ve_s-Ve_f;
    dXe_s_last(3)=0;
    dVe_s_last(3)=0;
end
if count == floor(Ts_gps/Ts)
    count = 1; 
    temp = ((Xe_s(1:2)-Xe_f(1:2)) + dXe_s_last(1:2) + dXe_s_last_2(1:2))/3;
    dXe_s_last_2 = dXe_s_last;
    dXe_s_last(1:2) = temp;
    dVe_s_last(1:2) = Ve_s(1:2)-Ve_f(1:2);
else
    count = count + 1;
end
Xe = Xe_f + dXe_s_last;
Ve = Ve_f + dVe_s_last;
Xe(3) = Xe_s(3);
Ve(3) = Ve_s(3);
